simulink model "lo_values_test_v2"  (R2012b)
settings: Solver=ode45  StartTime=0.0  StopTime=100000  RelTol=1e-3
values from neighbouring files (symbols this model uses):
  Fs = 640e6    (= 640000000)    [filter_coefficients.m]    (also in filter_design.m; filter_design_getting_order.m)
undefined symbols (not defined in the file or in its folder): get, sided, Two, xlipgetpartsetting
undefined symbols (not defined in the file): casper_coef
libraries: xbsIndex_r4 x608, dspsnks4 x18, dspsigops x8, dspspect3 x8, casper_library_misc x5, simulink x2, xps_library x1
(part 1 of 7)
settings Model: Creator=heystek  LastModifiedBy=heystek

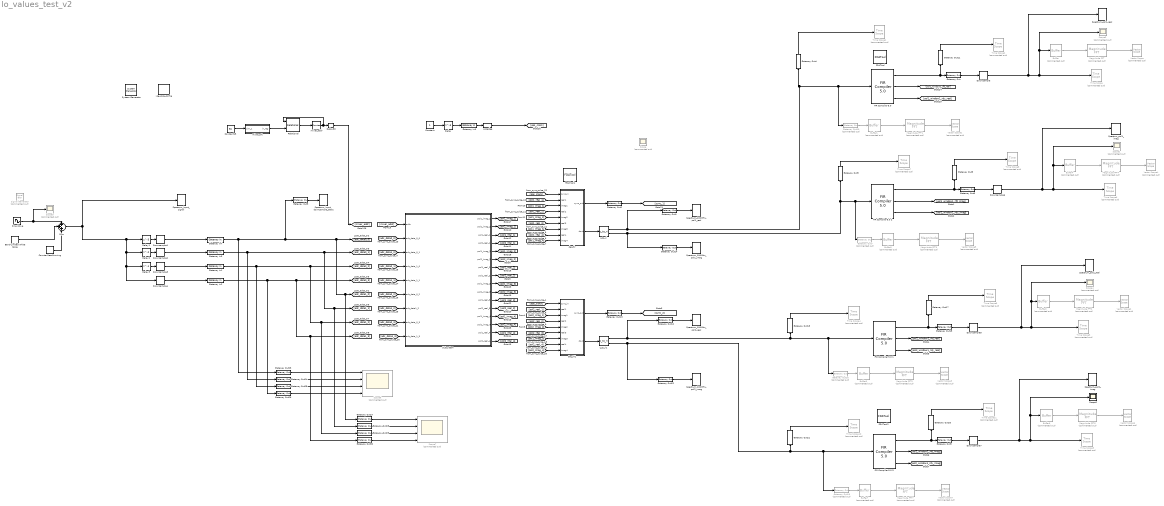
== system lo_values_test_v2 ==
  " System Generator" : xbsIndex_r4/ System Generator  Tag=genX  xilinxfamily=virtex6  part=xc6vsx475t  speed=-1  package=ff1759  synthesis_tool=XST  clock_wrapper=Clock Enables  directory=./window_design/sysgen  proj_type=Project Navigator  Synth_file=XST Defaults  Impl_file=ISE Defaults  testbench=off  simulink_period=1  sysclk_period=6.25  dcm_input_clock_period=100  incr_netlist=off  trim_vbits=Everywhere in SubSystem  dbl_ovrd=According to Block Masks  core_generation=According to Block Masks  run_coregen=off  deprecated_control=off  eval_field=0  block_type=sysgen
  Band-Limited White Noise : simulink/Sources/Band-Limited White Noise  Cov=[0.01]  Ts=0.25  seed=[23341]
  Buffer{,2,4,6} (4 alike) : Buffer  Commented=on  N=256  ic=20  TreatMby1Signals=One channel
  Buffer{1,3,5,7} (4 alike) : Buffer  Commented=on  N=1024  TreatMby1Signals=One channel
  Constant : Constant
  Constant15 : Constant  Value=61
  Counter Free-Running : simulink/Sources/Counter Free-Running  NumBits=8  tsamp=1
  Delay : Delay  DelayLength=3
  Delay1 : Delay  DelayLength=3
  Delay2 : Delay
  Delay3 : Delay  DelayLength=1
  Delay80 : xbsIndex_r4/Delay  rst=off  infoeditControl=Selection of Reset will increase slice count due to use of real FFs and instead of SRLs  en=off  latency=2  dbl_ovrd=off  reg_retiming=on  block_type=delay
      settings: block_version=11.4
  Downsample{,5..7} (4 alike) : dspsigops/Downsample  N=50  phase=0  RateOptions=Allow multirate processing  smode=Allow multirate  fmode=Maintain input frame size  ic=0
  Downsample{1..4} (4 alike) : dspsigops/Downsample  N=4  phase=0  RateOptions=Enforce single-rate processing  smode=Allow multirate  fmode=Maintain input frame size  ic=0
  FDATool : xbsIndex_r4/FDATool  block_type=fdatool
      settings: infoedit=FDATool
  FDATool1 : xbsIndex_r4/FDATool  block_type=fdatool
      settings: infoedit=FDATool
  FDATool2 : xbsIndex_r4/FDATool  block_type=fdatool
      settings: infoedit=FDATool
  "FIR Compiler 5.0 " : xbsIndex_r4/FIR Compiler 5.0   coefficientvector=coef  coefficient_sets=1  filter_type=Decimation  rate_change_type=Integer  interpolation_rate=1  decimation_rate=50  zero_pack_factor=1  number_channels=1  ratespecification=Maximum_Possible  sampleperiod=1  hardwareoversamplingrate=1  filter_architecture=Systolic_Multiply_Accumulate  coefficient_reload=off  coefficient_structure=Non_Symmetric  coefficient_sign=Unsigned  quantization=Maximize_Dynamic_Range  coefficient_width=25  bestprecision=on  coefficient_fractional_bits=33  number_paths=1  output_rounding_mode=Convergent_Rounding_to_Even  output_width=18  allow_rounding_approximation=off  optimization_goal=Area  has_sclr=off  has_data_valid=off  has_nd=off  has_ce=off  usechan_in_adv=off  chan_in_adv=0  data_buffer_type=Automatic  coefficient_buffer_type=Automatic  input_buffer_type=Automatic  output_buffer_type=Automatic  preference_for_other_storage=Automatic  multi_column_support=Disabled  columnconfig='12'  inter_column_pipe_length=4  passband_min=0.0  passband_max=0.5  stopband_min=0.5  stopband_max=1.0  filter_selection=1  gui_behaviour=Sysgen  registered_output=true  data_sign=Signed  data_width=16  data_fractional_bits=0  wrapper_available=true  ip_wrap_arbitrary_binary_point=true  ip_name=FIR Compiler  ip_version=5.0  dsptool_ready=true  ipcore_usecache=true  ipcore_useipmodelcache=true  ipcore_xco_need_fpga_part=true  port_translation_map={ 'ce' => 'en', 'sclr' => 'rst' }  run_core_at_system_period=true  ipcore_fpga_part=xlipgetpartsetting(gcb, {'virtex4', 'xc4vsx35', '-10', 'ff668'})  structural_sim=false  block_type=fir_compiler_v5_0
  FIR Compiler 5.0 1 : xbsIndex_r4/FIR Compiler 5.0   coefficientvector=coef  coefficient_sets=1  filter_type=Decimation  rate_change_type=Integer  interpolation_rate=1  decimation_rate=50  zero_pack_factor=1  number_channels=1  ratespecification=Maximum_Possible  sampleperiod=1  hardwareoversamplingrate=1  filter_architecture=Systolic_Multiply_Accumulate  coefficient_reload=off  coefficient_structure=Non_Symmetric  coefficient_sign=Unsigned  quantization=Maximize_Dynamic_Range  coefficient_width=25  bestprecision=on  coefficient_fractional_bits=35  number_paths=1  output_rounding_mode=Convergent_Rounding_to_Even  output_width=18  allow_rounding_approximation=off  optimization_goal=Area  has_sclr=off  has_data_valid=off  has_nd=off  has_ce=off  usechan_in_adv=off  chan_in_adv=0  data_buffer_type=Automatic  coefficient_buffer_type=Automatic  input_buffer_type=Automatic  output_buffer_type=Automatic  preference_for_other_storage=Automatic  multi_column_support=Disabled  columnconfig='42'  inter_column_pipe_length=4  passband_min=0.0  passband_max=0.5  stopband_min=0.5  stopband_max=1.0  filter_selection=1  gui_behaviour=Sysgen  registered_output=true  data_sign=Signed  data_width=16  data_fractional_bits=0  wrapper_available=true  ip_wrap_arbitrary_binary_point=true  ip_name=FIR Compiler  ip_version=5.0  dsptool_ready=true  ipcore_usecache=true  ipcore_useipmodelcache=true  ipcore_xco_need_fpga_part=true  port_translation_map={ 'ce' => 'en', 'sclr' => 'rst' }  run_core_at_system_period=true  ipcore_fpga_part=xlipgetpartsetting(gcb, {'virtex4', 'xc4vsx35', '-10', 'ff668'})  structural_sim=false  block_type=fir_compiler_v5_0
  FIR Compiler 5.0 2 : xbsIndex_r4/FIR Compiler 5.0   coefficientvector=coef  coefficient_sets=1  filter_type=Decimation  rate_change_type=Integer  interpolation_rate=1  decimation_rate=50  zero_pack_factor=1  number_channels=1  ratespecification=Maximum_Possible  sampleperiod=1  hardwareoversamplingrate=1  filter_architecture=Systolic_Multiply_Accumulate  coefficient_reload=off  coefficient_structure=Non_Symmetric  coefficient_sign=Unsigned  quantization=Maximize_Dynamic_Range  coefficient_width=25  bestprecision=on  coefficient_fractional_bits=33  number_paths=1  output_rounding_mode=Convergent_Rounding_to_Even  output_width=18  allow_rounding_approximation=off  optimization_goal=Area  has_sclr=off  has_data_valid=off  has_nd=off  has_ce=off  usechan_in_adv=off  chan_in_adv=0  data_buffer_type=Automatic  coefficient_buffer_type=Automatic  input_buffer_type=Automatic  output_buffer_type=Automatic  preference_for_other_storage=Automatic  multi_column_support=Disabled  columnconfig='12'  inter_column_pipe_length=4  passband_min=0.0  passband_max=0.5  stopband_min=0.5  stopband_max=1.0  filter_selection=1  gui_behaviour=Sysgen  registered_output=true  data_sign=Signed  data_width=16  data_fractional_bits=0  wrapper_available=true  ip_wrap_arbitrary_binary_point=true  ip_name=FIR Compiler  ip_version=5.0  dsptool_ready=true  ipcore_usecache=true  ipcore_useipmodelcache=true  ipcore_xco_need_fpga_part=true  port_translation_map={ 'ce' => 'en', 'sclr' => 'rst' }  run_core_at_system_period=true  ipcore_fpga_part=xlipgetpartsetting(gcb, {'virtex4', 'xc4vsx35', '-10', 'ff668'})  structural_sim=false  block_type=fir_compiler_v5_0
  FIR Compiler 5.0 3 : xbsIndex_r4/FIR Compiler 5.0   coefficientvector=coef  coefficient_sets=1  filter_type=Decimation  rate_change_type=Integer  interpolation_rate=1  decimation_rate=50  zero_pack_factor=1  number_channels=1  ratespecification=Maximum_Possible  sampleperiod=1  hardwareoversamplingrate=1  filter_architecture=Systolic_Multiply_Accumulate  coefficient_reload=off  coefficient_structure=Non_Symmetric  coefficient_sign=Unsigned  quantization=Maximize_Dynamic_Range  coefficient_width=25  bestprecision=on  coefficient_fractional_bits=33  number_paths=1  output_rounding_mode=Convergent_Rounding_to_Even  output_width=18  allow_rounding_approximation=off  optimization_goal=Area  has_sclr=off  has_data_valid=off  has_nd=off  has_ce=off  usechan_in_adv=off  chan_in_adv=0  data_buffer_type=Automatic  coefficient_buffer_type=Automatic  input_buffer_type=Automatic  output_buffer_type=Automatic  preference_for_other_storage=Automatic  multi_column_support=Disabled  columnconfig='12'  inter_column_pipe_length=4  passband_min=0.0  passband_max=0.5  stopband_min=0.5  stopband_max=1.0  filter_selection=1  gui_behaviour=Sysgen  registered_output=true  data_sign=Signed  data_width=16  data_fractional_bits=0  wrapper_available=true  ip_wrap_arbitrary_binary_point=true  ip_name=FIR Compiler  ip_version=5.0  dsptool_ready=true  ipcore_usecache=true  ipcore_useipmodelcache=true  ipcore_xco_need_fpga_part=true  port_translation_map={ 'ce' => 'en', 'sclr' => 'rst' }  run_core_at_system_period=true  ipcore_fpga_part=xlipgetpartsetting(gcb, {'virtex4', 'xc4vsx35', '-10', 'ff668'})  structural_sim=false  block_type=fir_compiler_v5_0
  Gateway In{1..3,7} (4 alike) : xbsIndex_r4/Gateway In  gui_display_data_type=Fixed-point  arith_type="Signed  (2's comp)"  n_bits=16  bin_pt=15  preci_type=Single  exp_width=8  frac_width=24  quantization="Round  (unbiased: +/- Inf)"  overflow=Saturate  period=1  dbl_ovrd=off  timing_constraint=None  locs_specified=off  LOCs={}  UseAsADC=off  ADCChannel='1'  inherit_from_input=off  hdl_port=on  block_type=gatewayin
  Gateway In5 : xbsIndex_r4/Gateway In  gui_display_data_type=Boolean  arith_type=Boolean  n_bits=16  bin_pt=15  preci_type=Single  exp_width=8  frac_width=24  quantization="Round  (unbiased: +/- Inf)"  overflow=Saturate  period=1  dbl_ovrd=off  timing_constraint=None  locs_specified=off  LOCs={}  UseAsADC=off  ADCChannel='1'  inherit_from_input=off  hdl_port=on  block_type=gatewayin
  Gateway Out{,5..6,15} (4 alike) : xbsIndex_r4/Gateway Out  inherit_from_input=on  hdl_port=off  timing_constraint=None  locs_specified=off  LOCs={}  UseAsDAC=off  DACChannel='1'  block_type=gatewayout
  Gateway Out{1..2,4,8..9,11..14,17..18,20..22,30} (15 alike) : xbsIndex_r4/Gateway Out  inherit_from_input=off  hdl_port=on  timing_constraint=None  locs_specified=off  LOCs={}  UseAsDAC=off  DACChannel='1'  block_type=gatewayout
  Gateway Out{7,10,16,19} (4 alike) : xbsIndex_r4/Gateway Out  Commented=on  inherit_from_input=off  hdl_port=on  timing_constraint=None  locs_specified=off  LOCs={}  UseAsDAC=off  DACChannel='1'  block_type=gatewayout
  Gateway Out{3,23..29} (8 alike) : xbsIndex_r4/Gateway Out  inherit_from_input=on  hdl_port=on  timing_constraint=None  locs_specified=off  LOCs={}  UseAsDAC=off  DACChannel='1'  block_type=gatewayout
  Magnitude FFT{,2,4,6} (4 alike) : dspspect3/Magnitude FFT  Commented=on  mag_or_magsq=Magnitude squared  FFTImplementation=Auto  fftLenInherit=off  fftsize=256
  Magnitude FFT{1,3,5,7} (4 alike) : dspspect3/Magnitude FFT  Commented=on  mag_or_magsq=Magnitude squared  FFTImplementation=Auto  fftLenInherit=off  fftsize=1024
  Relational : xbsIndex_r4/Relational  mode=a=b  en=off  latency=1  dbl_ovrd=off  block_type=relational
  Scope{,1,3..5} (5 alike) : Scope  Commented=on
      Scope1 settings: YMin=-0.00065  YMax=0.0002
      Scope3 settings: YMin=-0.00065  YMax=0.0002  SaveName=ScopeData3
      Scope4 settings: YMin=-0.00065  YMax=0.0002  SaveName=ScopeData4
      Scope5 settings: SaveName=ScopeData5  MaxDataPoints=10
  Scope2 : Scope
      settings: YMin=-0.00065  YMax=0.0002  SaveName=ScopeData2
  Scope6 : Scope  Commented=on  NumInputPorts=4
      settings: YMin=-5~-5~-5~-5  YMax=5~5~5~5  SaveName=ScopeData6
  Scope7 : Scope  Commented=on  NumInputPorts=4
      settings: YMin=-5~-5~-5~-5  YMax=5~5~5~5  SaveName=ScopeData7
  Signal Generator : SignalGenerator  Commented=on  Amplitude=0.1  Frequency=0.00353  VectorParams1D=off
  Sine Wave : Sin  SineType=Sample based  Amplitude=0.1  Frequency=5  Samples=2000  SampleTime=0.25  Offset=1
  Spectrum_100MHz_pol1_imag : dspsnks4/Spectrum Scope  ScopeProperties=on  Domain=Frequency  HorizSpan=1  UseBuffer=on  BufferSize=2^13  Overlap=0  TreatMby1Signals=One channel  inpFftLenInherit=on  FFTlength=2^13  numAvg=1  DisplayProperties=off  AxisGrid=on  Memory=off  FrameNumber=on  AxisLegend=off  AxisZoom=off  OpenScopeAtSimStart=on  OpenScopeImmediately=off  FigPos=get(0,'defaultfigureposition')  AxisProperties=off  XUnits=Hertz  XRange=Two-sided ((-Fs/2...Fs/2])  XDisplay=0  InheritXIncr=on  XIncr=1.0  XLabel=Samples  XLimit=Auto  YUnits=dBm/Hertz  XMax=1  XMin=0  YLabel=Magnitude-squared, dB  LineProperties=off  wintypeSpecScope=Hann  RsSpecScope=50  betaSpecScope=5  winsampSpecScope=Periodic  XAxisParamsVer=6.9  isFrameUpgraded=on
      settings: YMin=-10  YMax=10
  Spectrum_100MHz_pol1_real : dspsnks4/Spectrum Scope  ScopeProperties=on  Domain=Frequency  HorizSpan=1  UseBuffer=on  BufferSize=2^13  Overlap=0  TreatMby1Signals=One channel  inpFftLenInherit=on  FFTlength=2^13  numAvg=1  DisplayProperties=off  AxisGrid=on  Memory=off  FrameNumber=on  AxisLegend=off  AxisZoom=off  OpenScopeAtSimStart=on  OpenScopeImmediately=off  FigPos=get(0,'defaultfigureposition')  AxisProperties=off  XUnits=Hertz  XRange=Two-sided ((-Fs/2...Fs/2])  XDisplay=0  InheritXIncr=on  XIncr=1.0  XLabel=Samples  XLimit=Auto  YUnits=dBm/Hertz  XMax=1  XMin=0  YLabel=Magnitude-squared, dB  LineProperties=off  wintypeSpecScope=Hann  RsSpecScope=50  betaSpecScope=5  winsampSpecScope=Periodic  XAxisParamsVer=6.9  isFrameUpgraded=on
      settings: YMin=-10  YMax=10
  Spectrum_100MHz_pol2_imag : dspsnks4/Spectrum Scope  ScopeProperties=on  Domain=Frequency  HorizSpan=1  UseBuffer=on  BufferSize=2^13  Overlap=0  TreatMby1Signals=One channel  inpFftLenInherit=on  FFTlength=2^13  numAvg=5  DisplayProperties=off  AxisGrid=on  Memory=off  FrameNumber=on  AxisLegend=off  AxisZoom=off  OpenScopeAtSimStart=on  OpenScopeImmediately=off  FigPos=get(0,'defaultfigureposition')  AxisProperties=off  XUnits=Hertz  XRange=Two-sided ((-Fs/2...Fs/2])  XDisplay=0  InheritXIncr=on  XIncr=1.0  XLabel=Samples  XLimit=Auto  YUnits=dBm/Hertz  XMax=1  XMin=0  YLabel=Magnitude-squared, dB  LineProperties=off  wintypeSpecScope=Hann  RsSpecScope=50  betaSpecScope=5  winsampSpecScope=Periodic  XAxisParamsVer=6.9  isFrameUpgraded=on
      settings: YMin=-10  YMax=10
  Spectrum_100MHz_pol2_real : dspsnks4/Spectrum Scope  ScopeProperties=on  Domain=Frequency  HorizSpan=1  UseBuffer=on  BufferSize=2^13  Overlap=0  TreatMby1Signals=One channel  inpFftLenInherit=on  FFTlength=2^13  numAvg=1  DisplayProperties=off  AxisGrid=on  Memory=off  FrameNumber=on  AxisLegend=off  AxisZoom=off  OpenScopeAtSimStart=on  OpenScopeImmediately=off  FigPos=get(0,'defaultfigureposition')  AxisProperties=off  XUnits=Hertz  XRange=Two-sided ((-Fs/2...Fs/2])  XDisplay=0  InheritXIncr=on  XIncr=1.0  XLabel=Samples  XLimit=Auto  YUnits=dBm/Hertz  XMax=1  XMin=0  YLabel=Magnitude-squared, dB  LineProperties=off  wintypeSpecScope=Hann  RsSpecScope=50  betaSpecScope=5  winsampSpecScope=Periodic  XAxisParamsVer=6.9  isFrameUpgraded=on
      settings: YMin=-10  YMax=10
  Spectrum_input_downsample_delay : dspsnks4/Spectrum Scope  ScopeProperties=on  Domain=Frequency  HorizSpan=1  UseBuffer=on  BufferSize=2^15  Overlap=0  TreatMby1Signals=One channel  inpFftLenInherit=on  FFTlength=2^15  numAvg=5  DisplayProperties=off  AxisGrid=on  Memory=off  FrameNumber=on  AxisLegend=off  AxisZoom=off  OpenScopeAtSimStart=on  OpenScopeImmediately=off  FigPos=get(0,'defaultfigureposition')  AxisProperties=off  XUnits=Hertz  XRange=Two-sided ((-Fs/2...Fs/2])  XDisplay=0  InheritXIncr=on  XIncr=1.0  XLabel=Samples  XLimit=Auto  YUnits=dBW/Hertz  XMax=1  XMin=0  YLabel=Magnitude-squared, dB  LineProperties=off  wintypeSpecScope=Hann  RsSpecScope=50  betaSpecScope=5  winsampSpecScope=Periodic  XAxisParamsVer=6.9  isFrameUpgraded=on
      settings: YMin=-10  YMax=10
  Spectrum_input_signal : dspsnks4/Spectrum Scope  ScopeProperties=on  Domain=Frequency  HorizSpan=1  UseBuffer=on  BufferSize=2^15  Overlap=0  TreatMby1Signals=One channel  inpFftLenInherit=on  FFTlength=2^15  numAvg=1  DisplayProperties=off  AxisGrid=on  Memory=off  FrameNumber=on  AxisLegend=off  AxisZoom=off  OpenScopeAtSimStart=on  OpenScopeImmediately=off  FigPos=get(0,'defaultfigureposition')  AxisProperties=off  XUnits=Hertz  XRange=Two-sided ((-Fs/2...Fs/2])  XDisplay=0  InheritXIncr=on  XIncr=1.0  XLabel=Samples  XLimit=Auto  YUnits=dBW/Hertz  XMax=1  XMin=0  YLabel=Magnitude-squared, dB  LineProperties=off  wintypeSpecScope=Hann  RsSpecScope=50  betaSpecScope=5  winsampSpecScope=Periodic  XAxisParamsVer=6.9  isFrameUpgraded=on
      settings: YMin=-10  YMax=10
  Spectrum_pol1_real : dspsnks4/Spectrum Scope  ScopeProperties=on  Domain=Frequency  HorizSpan=1  UseBuffer=on  BufferSize=256  Overlap=0  TreatMby1Signals=One channel  inpFftLenInherit=on  FFTlength=256  numAvg=5  DisplayProperties=off  AxisGrid=on  Memory=off  FrameNumber=on  AxisLegend=off  AxisZoom=off  OpenScopeAtSimStart=on  OpenScopeImmediately=off  FigPos=get(0,'defaultfigureposition')  AxisProperties=off  XUnits=Hertz  XRange=Two-sided ((-Fs/2...Fs/2])  XDisplay=0  InheritXIncr=on  XIncr=1.0  XLabel=Samples  XLimit=Auto  YUnits=dBW/Hertz  XMax=1  XMin=0  YLabel=Magnitude-squared, dB  LineProperties=off  wintypeSpecScope=Hann  RsSpecScope=50  betaSpecScope=5  winsampSpecScope=Periodic  XAxisParamsVer=6.9  isFrameUpgraded=on
      settings: YMin=-10  YMax=10
  Spectrum_pol2_imag : dspsnks4/Spectrum Scope  ScopeProperties=on  Domain=Frequency  HorizSpan=1  UseBuffer=on  BufferSize=256  Overlap=0  TreatMby1Signals=One channel  inpFftLenInherit=on  FFTlength=256  numAvg=5  DisplayProperties=off  AxisGrid=on  Memory=off  FrameNumber=on  AxisLegend=off  AxisZoom=off  OpenScopeAtSimStart=on  OpenScopeImmediately=off  FigPos=get(0,'defaultfigureposition')  AxisProperties=off  XUnits=Hertz  XRange=Two-sided ((-Fs/2...Fs/2])  XDisplay=0  InheritXIncr=on  XIncr=1.0  XLabel=Samples  XLimit=Auto  YUnits=dBW/Hertz  XMax=1  XMin=0  YLabel=Magnitude-squared, dB  LineProperties=off  wintypeSpecScope=Hann  RsSpecScope=50  betaSpecScope=5  winsampSpecScope=Periodic  XAxisParamsVer=6.9  isFrameUpgraded=on
      settings: YMin=-10  YMax=10
  Spectrum_pol2_real : dspsnks4/Spectrum Scope  ScopeProperties=on  Domain=Frequency  HorizSpan=1  UseBuffer=on  BufferSize=256  Overlap=0  TreatMby1Signals=One channel  inpFftLenInherit=on  FFTlength=256  numAvg=5  DisplayProperties=off  AxisGrid=on  Memory=off  FrameNumber=on  AxisLegend=off  AxisZoom=off  OpenScopeAtSimStart=on  OpenScopeImmediately=off  FigPos=get(0,'defaultfigureposition')  AxisProperties=off  XUnits=Hertz  XRange=Two-sided ((-Fs/2...Fs/2])  XDisplay=0  InheritXIncr=on  XIncr=1.0  XLabel=Samples  XLimit=Auto  YUnits=dBW/Hertz  XMax=1  XMin=0  YLabel=Magnitude-squared, dB  LineProperties=off  wintypeSpecScope=Hann  RsSpecScope=50  betaSpecScope=5  winsampSpecScope=Periodic  XAxisParamsVer=6.9  isFrameUpgraded=on
      settings: YMin=-10  YMax=10
  Spectum_pol1_imag : dspsnks4/Spectrum Scope  ScopeProperties=on  Domain=Frequency  HorizSpan=1  UseBuffer=on  BufferSize=256  Overlap=0  TreatMby1Signals=One channel  inpFftLenInherit=on  FFTlength=256  numAvg=5  DisplayProperties=off  AxisGrid=on  Memory=off  FrameNumber=on  AxisLegend=off  AxisZoom=off  OpenScopeAtSimStart=on  OpenScopeImmediately=off  FigPos=get(0,'defaultfigureposition')  AxisProperties=off  XUnits=Hertz  XRange=Two-sided ((-Fs/2...Fs/2])  XDisplay=0  InheritXIncr=on  XIncr=1.0  XLabel=Samples  XLimit=Auto  YUnits=dBW/Hertz  XMax=1  XMin=0  YLabel=Magnitude-squared, dB  LineProperties=off  wintypeSpecScope=Hann  RsSpecScope=50  betaSpecScope=5  winsampSpecScope=Periodic  XAxisParamsVer=6.9  isFrameUpgraded=on
      settings: YMin=-10  YMax=10
  Subsystem : Subsystem
  Sum : Sum  Inputs=+++
  Time Scope{,1..11} (12 alike) : TimeScope  Commented=on  DefaultConfigurationName=spbscopes.TimeScopeBlockCfg
      settings: CopyFcn=scopeextensions.ScopeBlock.callback(gcbh, 'onBlockCopy', gcbh);  DeleteFcn=scopeextensions.ScopeBlock.callback(gcbh, 'onBlockDelete');  PreSaveFcn=scopeextensions.ScopeBlock.callback(gcbh, 'onModelSave');  NameChangeFcn=scopeextensions.ScopeBlock.callback(gcbh, 'onBlockRename');  OpenFcn=scopeextensions.SrcWiredSL.coreBlockCommand('Open',gcbh)  CloseFcn=scopeextensions.ScopeBlock.callback(gcbh, 'onBlockClose');  PreDeleteFcn=scopeextensions.ScopeBlock.callback(gcbh, 'onBlockPreDelete');
  Vector Scope{,2,4,6} (4 alike) : dspsnks4/Vector Scope  Commented=on  ScopeProperties=on  Domain=Frequency  HorizSpan=1  DisplayProperties=off  AxisGrid=on  Memory=off  FrameNumber=on  AxisLegend=on  AxisZoom=off  OpenScopeAtSimStart=on  OpenScopeImmediately=off  FigPos=get(0,'defaultfigureposition')  AxisProperties=off  XUnits=Hertz  XRange=[-Fs/2...Fs/2]  InheritXIncr=on  XIncr=50  XLabel=Time  XLimit=Auto  XMin=-1e6  XMax=1e6  XStart=0  YUnits=dB  YLabel=Amplitude  LineProperties=off  XAxisParamsVer=6.9
      settings: YMin=-50  YMax=30
  Vector Scope{1,3,5,7} (4 alike) : dspsnks4/Vector Scope  Commented=on  ScopeProperties=on  Domain=Frequency  HorizSpan=1  DisplayProperties=off  AxisGrid=on  Memory=off  FrameNumber=on  AxisLegend=on  AxisZoom=off  OpenScopeAtSimStart=on  OpenScopeImmediately=off  FigPos=get(0,'defaultfigureposition')  AxisProperties=off  XUnits=Hertz  XRange=[-Fs/2...Fs/2]  InheritXIncr=on  XIncr=1  XLabel=Time  XLimit=Auto  XMin=-1e6  XMax=1e6  XStart=0  YUnits=Magnitude  YLabel=Amplitude  LineProperties=off  XAxisParamsVer=6.9
      settings: YMin=-10  YMax=10
  c_to_ri : casper_library_misc/c_to_ri  n_bits=16  bin_pt=15
      settings: AttributesFormatString=16_15 r/i
  c_to_ri1 : casper_library_misc/c_to_ri  n_bits=16  bin_pt=15
      settings: AttributesFormatString=16_15 r/i
  dec_fir : Subsystem  Tag=casper:dec_fir  AncestorBlock=casper_library_downconverter/dec_fir  mask(dec_fir){n_inputs=4, coeff=casper_coef, n_bits=16, n_bits_bp=15, quantization=Round  (unbiased: +/- Inf), add_latency=1, mult_latency=2, conv_latency=2, coeff_bit_width=25, coeff_bin_pt=24, absorb_adders=on, adder_imp=DSP48, lshift=1}
      mask prompts: n_inputs "Number of Parallel Streams"; coeff "Coefficients"; n_bits "Bit Width Out"; n_bits_bp "Bin Pt Out"; quantization "Quantization Behavior"; add_latency "Add Latency"; mult_latency "Mult Latency"; conv_latency "Convert latency"; coeff_bit_width "Coefficient bit width"; coeff_bin_pt "Coefficient binary point"; absorb_adders "Absorb adders into DSP slices"; adder_imp "Adder implementation"; lshift "Post adder-tree shift"
      mask help: FIR filter which can handle multiple time samples in parallel and decimates down to 1 time sample. If coefficients are symmetric, will automatically fold before multiplying.
      mask init:
      | dec_fir_init(gcb, ...
      |     'n_inputs', n_inputs, ...
      |     'coeff', coeff, ...
      |     'n_bits', n_bits, ...
      |     'n_bits_bp', n_bits_bp, ...
      |     'quantization', quantization, ...
      |     'add_latency', add_latency, ...
      |     'mult_latency', mult_latency, ...
      |     'conv_latency', conv_latency, ...
      |     'coeff_bit_width', coeff_bit_width, ...
      |     'coeff_bin_pt', coeff_bin_pt, ...
      |     'absorb_adders', absorb_adders, ...
      |     'adder_imp', adder_imp, ...
      |     'lshift', lshift);
      settings: AttributesFormatString=|
      | 16 taps
      | 16_15 r/i
      mask TypeOptions quantization: Truncate | Round  (unbiased: +/- Inf) | Round  (unbiased: Even Values)
      mask TypeOptions adder_imp: Behavioral | Fabric | DSP48
  dec_fir1 : Subsystem  Tag=casper:dec_fir  AncestorBlock=casper_library_downconverter/dec_fir  mask(dec_fir){n_inputs=4, coeff=casper_coef, n_bits=16, n_bits_bp=15, quantization=Round  (unbiased: +/- Inf), add_latency=1, mult_latency=2, conv_latency=2, coeff_bit_width=25, coeff_bin_pt=24, absorb_adders=on, adder_imp=DSP48, lshift=1}
      mask prompts: n_inputs "Number of Parallel Streams"; coeff "Coefficients"; n_bits "Bit Width Out"; n_bits_bp "Bin Pt Out"; quantization "Quantization Behavior"; add_latency "Add Latency"; mult_latency "Mult Latency"; conv_latency "Convert latency"; coeff_bit_width "Coefficient bit width"; coeff_bin_pt "Coefficient binary point"; absorb_adders "Absorb adders into DSP slices"; adder_imp "Adder implementation"; lshift "Post adder-tree shift"
      mask help: FIR filter which can handle multiple time samples in parallel and decimates down to 1 time sample. If coefficients are symmetric, will automatically fold before multiplying.
      mask init: same as lo_values_test_v2/dec_fir
      settings: AttributesFormatString=|
      | 16 taps
      | 16_15 r/i
      mask TypeOptions quantization: Truncate | Round  (unbiased: +/- Inf) | Round  (unbiased: Even Values)
      mask TypeOptions adder_imp: Behavioral | Fabric | DSP48
  mixer_addr : xbsIndex_r4/Counter  cnt_type=Free Running  cnt_to=Inf  operation=Up  start_count=0  cnt_by_val=1  arith_type="Signed  (2's comp)"  n_bits=16  bin_pt=15  load_pin=off  rst=on  en=off  explicit_period=on  period=1  dbl_ovrd=off  use_behavioral_HDL=off  implementation=Fabric  block_type=counter
      settings: block_version=11.4
  mixer_cnt : Subsystem  Tag=xps:sw_reg  AncestorBlock=xps_library/software_register  mask(swreg){io_dir=From Processor, io_delay=0, sample_period=1, names=reg, bitwidths=32, bin_pts=0, arith_types=0, sim_port=on, show_format=on}
      mask prompts: io_dir "I/O direction"; io_delay "I/O delay"; sample_period "Sample period"; names "Bitfield names [msb...lsb]"; bitwidths "Bitfield widths"; bin_pts "Bitfield binary pts"; arith_types "Bitfield types, ufix=0, fix=1, bool=2"; sim_port "Provide sim input/output?"; show_format "Print format string?"
      mask help: A 32-bit software-accessible register. Can be divided into bitfields of varying widths and types using the fields in the block mask.
      mask init:
      | try
      |     swreg_init(gcb)
      | catch ex
      |     disp(sprintf('%s: %s', gcb, ex.message))
      |     errordlg(ex.message)
      | end
      settings: AttributesFormatString=1input:uf32.0 = 32 bits
      mask TypeOptions io_dir: To Processor | From Processor
      mask Callback io_dir:
      | mask_enables = get_param(gcb, 'MaskEnables');
      | mask_names = get_param(gcb, 'MaskNames');
      | if strcmp(get_param(gcb, 'io_dir'), 'To Processor'),
      |     mask_enables{ismember(mask_names, 'sample_period')} = 'off';
      | else
      |     mask_enables{ismember(mask_names, 'sample_period')} = 'on';
      | end
      | set_param(gcb, 'MaskEnables', mask_enables);
  posedge : casper_library_misc/posedge  Tag=Rising Edge Detector
  xsg_core_config : xps_library/XSG_core_config  Tag=xps:xsg  hw_sys=ROACH2:sx475t  clk_src=sys_clk  ROACH_clk_src=adc0_clk  ROACH2_clk_src=sys_clk  MKDIG_clk_src=sys_clk  clk_rate=200  sample_period=1  synthesis_tool=XST
  wires:
  Delay/1 -> Gateway In5/1
  Constant/1 -> Delay/1
  Gateway Out2/1 -> [sync_1]
  Gateway In5/1 -> posedge/1
  Downsample1/1 -> Gateway In7/1
  Band-Limited White Noise/1 -> Sum/2
  Sine Wave/1 -> Scope5/1, Sum/1
  Counter Free-Running/1 -> Sum/3
  Delay1/1 -> Downsample1/1
  Delay2/1 -> Downsample2/1
  Delay3/1 -> Downsample3/1
  "FIR Compiler 5.0 "/2 -> [pol1_window1_rfd_real]
  "FIR Compiler 5.0 "/3 -> [pol1_window1_rdy_real]
  c_to_ri/1 -> Gateway Out10/1, "FIR Compiler 5.0 "/1, Gateway Out4/1, Gateway Out1/1
  Gateway Out/1 -> Downsample/1
  Magnitude FFT/1 -> Vector Scope/1
  Magnitude FFT1/1 -> Vector Scope1/1
  Gateway Out10/1 -> Buffer1/1
  "FIR Compiler 5.0 "/1 -> Gateway Out/1, Gateway Out11/1
  Gateway Out11/1 -> Time Scope2/1
  dec_fir/1(sync_out) -> Gateway Out2/1
  posedge/1 -> [pps_clock]
  dec_fir/2(dout) -> c_to_ri/1
  mixer_addr/1 -> Relational/1, Delay80/1
  Delay80/1 -> [mixer_addr]
  Relational/1 -> mixer_addr/1
  mixer_cnt/1(in_reg) -> Relational/2
  Constant15/1 -> mixer_cnt/1(sim_1)
  [pps_clock] -> dec_fir/1(sync_in)
  [pol1_real_1] -> dec_fir/2(real1)
  [pol1_imag_1] -> dec_fir/3(imag1)
  [pol1_real_2] -> dec_fir/4(real2)
  [pol1_imag_2] -> dec_fir/5(imag2)
  [pol1_real_3] -> dec_fir/6(real3)
  [pol1_imag_3] -> dec_fir/7(imag3)
  [pol1_imag_4] -> dec_fir/9(imag4)
  [pol1_real_4] -> dec_fir/8(real4)
  Gateway Out13/1 -> [sync_2]
  dec_fir1/1(sync_out) -> Gateway Out13/1
  dec_fir1/2(dout) -> c_to_ri1/1
  [pps_clock] -> dec_fir1/1(sync_in)
  [pol2_real_1] -> dec_fir1/2(real1)
  [pol2_imag_1] -> dec_fir1/3(imag1)
  [pol2_real_2] -> dec_fir1/4(real2)
  [pol2_imag_2] -> dec_fir1/5(imag2)
  [pol2_real_3] -> dec_fir1/6(real3)
  [pol1_imag_3] -> dec_fir1/7(imag3)
  [pol2_imag_4] -> dec_fir1/9(imag4)
  [pol2_real_4] -> dec_fir1/8(real4)
  FIR Compiler 5.0 1/2 -> [pol2_window1_rfd_real]
  FIR Compiler 5.0 1/3 -> [pol2_window1_rdy_real]
  c_to_ri1/1 -> Gateway Out16/1, FIR Compiler 5.0 1/1, Gateway Out18/1, Gateway Out12/1
  Gateway Out15/1 -> Downsample5/1
  Magnitude FFT2/1 -> Vector Scope2/1
  Buffer3/1 -> Magnitude FFT3/1
  Magnitude FFT3/1 -> Vector Scope3/1
  Gateway Out16/1 -> Buffer3/1
  FIR Compiler 5.0 1/1 -> Gateway Out15/1, Gateway Out17/1
  Gateway Out17/1 -> Time Scope5/1
  Subsystem/1(pol1_imag_1) -> [pol1_imag_1]
  Subsystem/2(pol2_imag_2) -> [pol2_imag_1]
  Subsystem/3(pol1_real_1) -> [pol1_real_1]
  Subsystem/4(pol2_real_1) -> [pol2_real_1]
  Subsystem/5(pol1_imag_2) -> [pol1_imag_2]
  Subsystem/6("pol2_imag_2 ") -> [pol2_imag_2]
  Subsystem/7(pol1_real_2) -> [pol1_real_2]
  Subsystem/8(pol2_real_2) -> [pol2_real_2]
  Subsystem/9(pol1_imag_3) -> [pol1_imag_3]
  Subsystem/10(pol2_imag_3) -> [pol2_imag_3]
  Subsystem/11(pol1_real_3) -> [pol1_real_3]
  Subsystem/12(pol2_real_3) -> [pol2_real_3]
  Subsystem/13(pol1_imag_4) -> [pol1_imag_4]
  Subsystem/14(pol2_imag_4) -> [pol2_imag_4]
  Subsystem/15(pol1_real_4) -> [pol1_real_4]
  Subsystem/16(pol2_real_4) -> [pol2_real_4]
  [adc_data0_0] -> Subsystem/2(adc_data_0_0)
  [adc_data1_0] -> Subsystem/3(adc_data_0_1)
  [adc_data0_1] -> Subsystem/4(adc_data_1_0)
  [adc_data1_1] -> Subsystem/5(adc_data_1_1)
  [adc_data0_2] -> Subsystem/6(adc_data_0_2)
  [adc_data1_2] -> Subsystem/7(adc_data1_2)
  [adc_data0_3] -> Subsystem/8(adc_data_0_3)
  [adc_data1_3] -> Subsystem/9(adc_data_1_3)
  [mixer_addr] -> Subsystem/1(addr)
  Gateway Out1/1 -> Spectrum_100MHz_pol1_real/1
  Gateway Out12/1 -> Spectrum_100MHz_pol2_real/1
  Gateway Out4/1 -> Time Scope1/1
  Gateway Out18/1 -> Time Scope4/1
  Sum/1 -> Delay1/1, Delay2/1, Delay3/1, Downsample4/1, Spectrum_input_signal/1
  Downsample2/1 -> Gateway In3/1
  Downsample3/1 -> Gateway In1/1
  Downsample4/1 -> Gateway In2/1
  Gateway In7/1 -> Gateway Out23/1, Gateway Out3/1, Gateway Out27/1, [adc_data1_0], [adc_data0_0]
  Gateway In3/1 -> Gateway Out24/1, Gateway Out28/1, [adc_data1_1], [adc_data0_1]
  Gateway In2/1 -> Gateway Out26/1, Gateway Out30/1, [adc_data1_3], [adc_data0_3]
  Gateway Out3/1 -> Spectrum_input_downsample_delay/1
  Downsample/1 -> Spectrum_pol1_real/1, Scope3/1, Buffer/1, Time Scope/1
  Downsample5/1 -> Spectrum_pol2_real/1, Scope4/1, Buffer2/1, Time Scope3/1
  Buffer2/1 -> Magnitude FFT2/1
  Buffer/1 -> Magnitude FFT/1
  FIR Compiler 5.0 2/2 -> [pol1_window1_rfd_imag]
  FIR Compiler 5.0 2/3 -> [pol1_window1_rdy_imag]
  Gateway Out6/1 -> Downsample6/1
  Magnitude FFT4/1 -> Vector Scope4/1
  Magnitude FFT5/1 -> Vector Scope5/1
  Gateway Out7/1 -> Buffer5/1
  FIR Compiler 5.0 2/1 -> Gateway Out6/1, Gateway Out8/1
  Gateway Out8/1 -> Time Scope8/1
  Gateway Out9/1 -> Time Scope7/1
  Downsample6/1 -> Spectum_pol1_imag/1, Scope1/1, Buffer4/1, Time Scope6/1
  Buffer4/1 -> Magnitude FFT4/1
  Buffer1/1 -> Magnitude FFT1/1
  Buffer5/1 -> Magnitude FFT5/1
  FIR Compiler 5.0 3/2 -> [pol2_window1_rfd_imag]
  FIR Compiler 5.0 3/3 -> [pol2_window1_rdy_imag]
  Gateway Out5/1 -> Downsample7/1
  Magnitude FFT6/1 -> Vector Scope6/1
  Buffer7/1 -> Magnitude FFT7/1
  Magnitude FFT7/1 -> Vector Scope7/1
  Gateway Out19/1 -> Buffer7/1
  FIR Compiler 5.0 3/1 -> Gateway Out5/1, Gateway Out20/1
  Gateway Out20/1 -> Time Scope11/1
  Gateway Out21/1 -> Time Scope10/1
  Downsample7/1 -> Spectrum_pol2_imag/1, Scope2/1, Buffer6/1, Time Scope9/1
  Buffer6/1 -> Magnitude FFT6/1
  c_to_ri/2 -> Gateway Out14/1, Gateway Out9/1, Gateway Out7/1, FIR Compiler 5.0 2/1
  Gateway Out14/1 -> Spectrum_100MHz_pol1_imag/1
  c_to_ri1/2 -> Gateway Out22/1, Gateway Out21/1, Gateway Out19/1, FIR Compiler 5.0 3/1
  Gateway Out22/1 -> Spectrum_100MHz_pol2_imag/1
  Gateway Out23/1 -> Scope6/1
  Gateway Out24/1 -> Scope6/2
  Gateway Out25/1 -> Scope6/3
  Gateway Out26/1 -> Scope6/4
  Gateway In1/1 -> Gateway Out25/1, Gateway Out29/1, [adc_data1_2], [adc_data0_2]
  Gateway Out27/1 -> Scope7/1
  Gateway Out28/1 -> Scope7/2
  Gateway Out29/1 -> Scope7/3
  Gateway Out30/1 -> Scope7/4

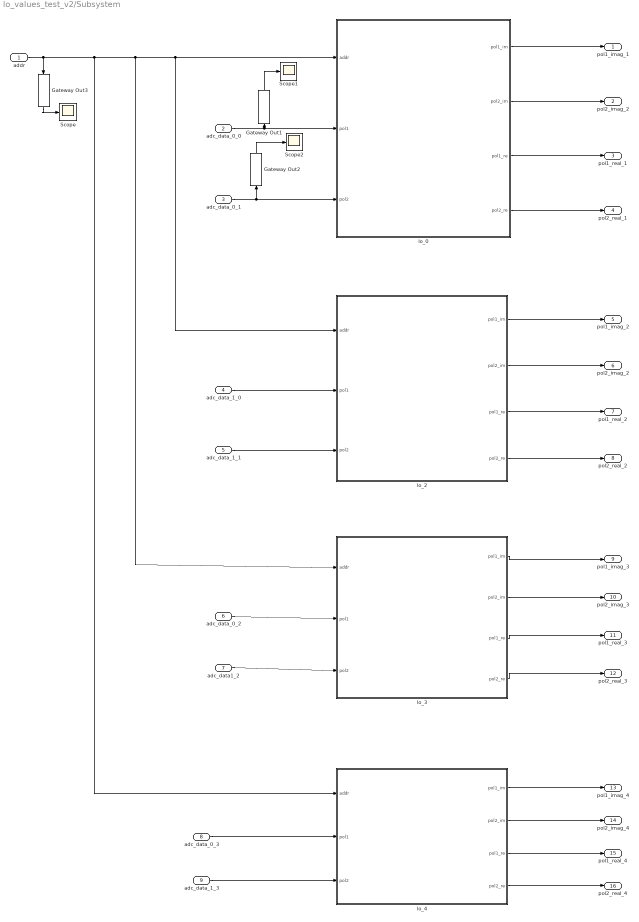
== system lo_values_test_v2/Subsystem ==
  addr : Inport
  adc_data_0_0 : Inport  Port=2
  adc_data_0_1 : Inport  Port=3
  adc_data_1_0 : Inport  Port=4
  adc_data_1_1 : Inport  Port=5
  adc_data_0_2 : Inport  Port=6
  adc_data1_2 : Inport  Port=7
  adc_data_0_3 : Inport  Port=8
  adc_data_1_3 : Inport  Port=9
  Gateway Out1 : xbsIndex_r4/Gateway Out  inherit_from_input=on  hdl_port=on  timing_constraint=None  locs_specified=off  LOCs={}  UseAsDAC=off  DACChannel='1'  block_type=gatewayout
  Gateway Out2 : xbsIndex_r4/Gateway Out  inherit_from_input=on  hdl_port=on  timing_constraint=None  locs_specified=off  LOCs={}  UseAsDAC=off  DACChannel='1'  block_type=gatewayout
  Gateway Out3 : xbsIndex_r4/Gateway Out  inherit_from_input=on  hdl_port=on  timing_constraint=None  locs_specified=off  LOCs={}  UseAsDAC=off  DACChannel='1'  block_type=gatewayout
  Scope : Scope
      settings: SaveName=ScopeData4
  Scope1 : Scope
      settings: YMin=-0.11  YMax=0.11  SaveName=ScopeData5
  Scope2 : Scope
      settings: YMin=-0.11  YMax=0.11  SaveName=ScopeData6
  lo_0 : Subsystem  AncestorBlock=gbt_library/complex_mix_lo
  lo_2 : Subsystem  AncestorBlock=gbt_library/complex_mix_lo
  lo_3 : Subsystem  AncestorBlock=gbt_library/complex_mix_lo
  lo_4 : Subsystem  AncestorBlock=gbt_library/complex_mix_lo
  pol1_imag_1 : Outport
  pol2_imag_2 : Outport  Port=2
  pol1_real_1 : Outport  Port=3
  pol2_real_1 : Outport  Port=4
  pol1_imag_2 : Outport  Port=5
  "pol2_imag_2 " : Outport  Port=6
  pol1_real_2 : Outport  Port=7
  pol2_real_2 : Outport  Port=8
  pol1_imag_3 : Outport  Port=9
  pol2_imag_3 : Outport  Port=10
  pol1_real_3 : Outport  Port=11
  pol2_real_3 : Outport  Port=12
  pol1_imag_4 : Outport  Port=13
  pol2_imag_4 : Outport  Port=14
  pol1_real_4 : Outport  Port=15
  pol2_real_4 : Outport  Port=16
  wires:
  lo_0/3(pol1_re) -> pol1_real_1/1
  lo_4/4(pol2_re) -> pol2_real_4/1
  adc_data_0_1/1 -> lo_0/3(pol2), Gateway Out2/1
  adc_data_1_0/1 -> lo_2/2(pol1)
  lo_4/3(pol1_re) -> pol1_real_4/1
  lo_4/2(pol2_im) -> pol2_imag_4/1
  adc_data_0_3/1 -> lo_4/2(pol1)
  lo_3/4(pol2_re) -> pol2_real_3/1
  adc_data_1_3/1 -> lo_4/3(pol2)
  lo_0/1(pol1_im) -> pol1_imag_1/1
  adc_data1_2/1 -> lo_3/3(pol2)
  lo_2/1(pol1_im) -> pol1_imag_2/1
  lo_0/4(pol2_re) -> pol2_real_1/1
  lo_2/3(pol1_re) -> pol1_real_2/1
  adc_data_0_0/1 -> lo_0/2(pol1), Gateway Out1/1
  lo_0/2(pol2_im) -> pol2_imag_2/1
  lo_4/1(pol1_im) -> pol1_imag_4/1
  adc_data_0_2/1 -> lo_3/2(pol1)
  lo_3/3(pol1_re) -> pol1_real_3/1
  adc_data_1_1/1 -> lo_2/3(pol2)
  lo_2/4(pol2_re) -> pol2_real_2/1
  addr/1 -> Gateway Out3/1, lo_4/1(addr), lo_2/1(addr), lo_0/1(addr), lo_3/1(addr)
  lo_3/1(pol1_im) -> pol1_imag_3/1
  lo_3/2(pol2_im) -> pol2_imag_3/1
  lo_2/2(pol2_im) -> "pol2_imag_2 "/1
  Gateway Out3/1 -> Scope/1
  Gateway Out1/1 -> Scope1/1
  Gateway Out2/1 -> Scope2/1

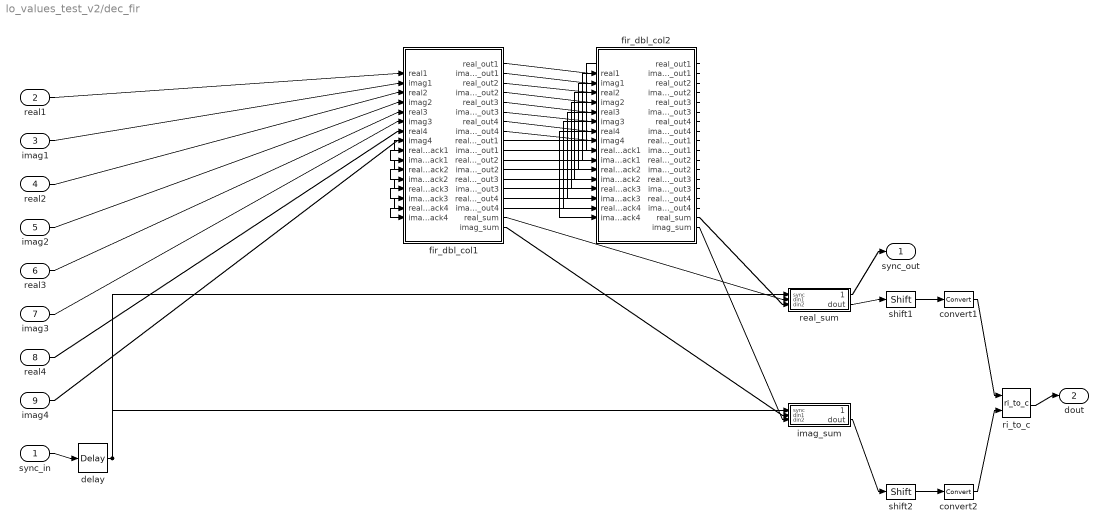
== system lo_values_test_v2/dec_fir ==
  sync_in : Inport
  real1 : Inport  Port=2
  imag1 : Inport  Port=3
  real2 : Inport  Port=4
  imag2 : Inport  Port=5
  real3 : Inport  Port=6
  imag3 : Inport  Port=7
  real4 : Inport  Port=8
  imag4 : Inport  Port=9
  convert1 : xbsIndex_r4/Convert  gui_display_data_type=Fixed-point  arith_type="Signed  (2's comp)"  n_bits=16  bin_pt=15  float_type=Single  exp_bits=8  fraction_bits=24  quantization="Round  (unbiased: +/- Inf)"  overflow=Wrap  en=off  latency=2  dbl_ovrd=off  pipeline=off  block_type=convert
  convert2 : xbsIndex_r4/Convert  gui_display_data_type=Fixed-point  arith_type="Signed  (2's comp)"  n_bits=16  bin_pt=15  float_type=Single  exp_bits=8  fraction_bits=24  quantization="Round  (unbiased: +/- Inf)"  overflow=Wrap  en=off  latency=2  dbl_ovrd=off  pipeline=off  block_type=convert
  delay : xbsIndex_r4/Delay  rst=off  infoeditControl=Selection of Reset will increase slice count due to use of real FFs and instead of SRLs  en=off  latency=7  dbl_ovrd=off  reg_retiming=off  block_type=delay
  fir_dbl_col1 : Subsystem  AncestorBlock=casper_library_downconverter/fir_dbl_col  mask(fir_dbl_col){n_inputs=4, coeff=[0.037109    0.023207    0.012354   0.0056253], add_latency=1, mult_latency=2, coeff_bit_width=25, coeff_bin_pt=24, first_stage_hdl=on, adder_imp=DSP48}
      mask prompts: n_inputs "Inputs"; coeff "Coefficients"; add_latency "Add latency"; mult_latency "Mult Latency"; coeff_bit_width "Coefficient bit width"; coeff_bin_pt "Coefficient binary point"; first_stage_hdl "Implement first stage of adder trees on output as behavioural HDL"; adder_imp "Adder implementation"
      mask init:
      | fir_dbl_col_init(gcb, ...
      |     'n_inputs', n_inputs, ...
      |     'coeff', coeff, ...
      |     'mult_latency', mult_latency, ...
      |     'add_latency', add_latency, ...
      |     'coeff_bit_width', coeff_bit_width, ...
      |     'coeff_bin_pt', coeff_bin_pt,  ...
      |     'first_stage_hdl', first_stage_hdl, ...
      |     'adder_imp', adder_imp);
      mask Help: eval('xlWeb(''http://casper.berkeley.edu/wiki/Fir_dbl_col'')')
      mask TypeOptions adder_imp: Behavioral | Fabric | DSP48
  fir_dbl_col2 : Subsystem  AncestorBlock=casper_library_downconverter/fir_dbl_col  mask(fir_dbl_col){n_inputs=4, coeff=[0.08556    0.079092    0.067391    0.052572], add_latency=1, mult_latency=2, coeff_bit_width=25, coeff_bin_pt=24, first_stage_hdl=on, adder_imp=DSP48}
      mask prompts: n_inputs "Inputs"; coeff "Coefficients"; add_latency "Add latency"; mult_latency "Mult Latency"; coeff_bit_width "Coefficient bit width"; coeff_bin_pt "Coefficient binary point"; first_stage_hdl "Implement first stage of adder trees on output as behavioural HDL"; adder_imp "Adder implementation"
      mask init: same as lo_values_test_v2/dec_fir/fir_dbl_col1
      mask Help: eval('xlWeb(''http://casper.berkeley.edu/wiki/Fir_dbl_col'')')
      mask TypeOptions adder_imp: Behavioral | Fabric | DSP48
  imag_sum : Subsystem  AncestorBlock=casper_library_misc/adder_tree  mask(adder_tree){n_inputs=2, latency=1, adder_imp=DSP48, first_stage_hdl=off}
      mask prompts: n_inputs "Number of Inputs"; latency "Add Latency"; adder_imp "Adder implementation"; first_stage_hdl "Use behavioural HDL for first stage of adders"
      mask help:
      | Sums all inputs using a tree of adds and delays.
      |
      | Number of inputs: The number of inputs to the block to be summed
      | Add latency: The number of clock cycles to perform one addition (affects timing)..
      | Adder implementation: choice of fabric or DSP48E core, or behavioral HDL
      | Use behavioural HDL for first stage of adders: Causes the first stage of adders to be absorbed into DSP blocks if multipliers precede them (Virtex 5). Overrides Adder implementation
      mask init:
      | adder_tree_init(gcb, ...
      |     'n_inputs', n_inputs, ...
      |     'latency', latency, ...
      |     'adder_imp', adder_imp, ...
      |     'first_stage_hdl', first_stage_hdl);
      settings: AttributesFormatString=latency 1
      mask Help: eval('xlWeb(''http://casper.berkeley.edu/wiki/Adder_tree'')')
      mask TypeOptions adder_imp: Behavioral | Fabric | DSP48
  real_sum : Subsystem  AncestorBlock=casper_library_misc/adder_tree  mask(adder_tree){n_inputs=2, latency=1, adder_imp=DSP48, first_stage_hdl=off}
      mask prompts: n_inputs "Number of Inputs"; latency "Add Latency"; adder_imp "Adder implementation"; first_stage_hdl "Use behavioural HDL for first stage of adders"
      mask help:
      | Sums all inputs using a tree of adds and delays.
      |
      | Number of inputs: The number of inputs to the block to be summed
      | Add latency: The number of clock cycles to perform one addition (affects timing)..
      | Adder implementation: choice of fabric or DSP48E core, or behavioral HDL
      | Use behavioural HDL for first stage of adders: Causes the first stage of adders to be absorbed into DSP blocks if multipliers precede them (Virtex 5). Overrides Adder implementation
      mask init:
      | adder_tree_init(gcb, ...
      |     'n_inputs', n_inputs, ...
      |     'latency', latency, ...
      |     'adder_imp', adder_imp, ...
      |     'first_stage_hdl', first_stage_hdl);
      settings: AttributesFormatString=latency 1
      mask Help: eval('xlWeb(''http://casper.berkeley.edu/wiki/Adder_tree'')')
      mask TypeOptions adder_imp: Behavioral | Fabric | DSP48
  ri_to_c : casper_library_misc/ri_to_c
  shift1 : xbsIndex_r4/Shift  shift_dir=Left  shift_bits=1  en=off  latency=0  precision=Full  arith_type="Signed  (2's comp)"  n_bits=16  bin_pt=14  quantization=Truncate  overflow=Wrap  dbl_ovrd=off  block_type=shift
  shift2 : xbsIndex_r4/Shift  shift_dir=Left  shift_bits=1  en=off  latency=0  precision=Full  arith_type="Signed  (2's comp)"  n_bits=16  bin_pt=14  quantization=Truncate  overflow=Wrap  dbl_ovrd=off  block_type=shift
  sync_out : Outport
  dout : Outport  Port=2
  wires:
  real1/1 -> fir_dbl_col1/1(real1)
  imag1/1 -> fir_dbl_col1/2(imag1)
  real2/1 -> fir_dbl_col1/3(real2)
  imag2/1 -> fir_dbl_col1/4(imag2)
  real3/1 -> fir_dbl_col1/5(real3)
  imag3/1 -> fir_dbl_col1/6(imag3)
  real4/1 -> fir_dbl_col1/7(real4)
  imag4/1 -> fir_dbl_col1/8(imag4)
  fir_dbl_col1/17(real_sum) -> real_sum/2(din1)
  fir_dbl_col1/18(imag_sum) -> imag_sum/2(din1)
  fir_dbl_col1/1(real_out1) -> fir_dbl_col2/1(real1)
  fir_dbl_col1/2(imag_out1) -> fir_dbl_col2/2(imag1)
  fir_dbl_col1/3(real_out2) -> fir_dbl_col2/3(real2)
  fir_dbl_col1/4(imag_out2) -> fir_dbl_col2/4(imag2)
  fir_dbl_col1/5(real_out3) -> fir_dbl_col2/5(real3)
  fir_dbl_col1/6(imag_out3) -> fir_dbl_col2/6(imag3)
  fir_dbl_col1/7(real_out4) -> fir_dbl_col2/7(real4)
  fir_dbl_col1/8(imag_out4) -> fir_dbl_col2/8(imag4)
  fir_dbl_col2/17(real_sum) -> real_sum/3(din2)
  fir_dbl_col2/18(imag_sum) -> imag_sum/3(din2)
  real_sum/2(dout) -> shift1/1
  imag_sum/2(dout) -> shift2/1
  shift1/1 -> convert1/1
  shift2/1 -> convert2/1
  convert1/1 -> ri_to_c/1
  convert2/1 -> ri_to_c/2
  ri_to_c/1 -> dout/1
  sync_in/1 -> delay/1
  delay/1 -> real_sum/1(sync), imag_sum/1(sync)
  real_sum/1(sync_out) -> sync_out/1
  fir_dbl_col2/9(real_back_out1) -> fir_dbl_col1/9(real_back1)
  fir_dbl_col2/10(imag_back_out1) -> fir_dbl_col1/10(imag_back1)
  fir_dbl_col2/11(real_back_out2) -> fir_dbl_col1/11(real_back2)
  fir_dbl_col2/12(imag_back_out2) -> fir_dbl_col1/12(imag_back2)
  fir_dbl_col2/13(real_back_out3) -> fir_dbl_col1/13(real_back3)
  fir_dbl_col2/14(imag_back_out3) -> fir_dbl_col1/14(imag_back3)
  fir_dbl_col2/15(real_back_out4) -> fir_dbl_col1/15(real_back4)
  fir_dbl_col2/16(imag_back_out4) -> fir_dbl_col1/16(imag_back4)
  fir_dbl_col2/1(real_out1) -> fir_dbl_col2/9(real_back1)
  fir_dbl_col2/2(imag_out1) -> fir_dbl_col2/10(imag_back1)
  fir_dbl_col2/3(real_out2) -> fir_dbl_col2/11(real_back2)
  fir_dbl_col2/4(imag_out2) -> fir_dbl_col2/12(imag_back2)
  fir_dbl_col2/5(real_out3) -> fir_dbl_col2/13(real_back3)
  fir_dbl_col2/6(imag_out3) -> fir_dbl_col2/14(imag_back3)
  fir_dbl_col2/7(real_out4) -> fir_dbl_col2/15(real_back4)
  fir_dbl_col2/8(imag_out4) -> fir_dbl_col2/16(imag_back4)
